simulink model "prescan_repl1"  (R2019a)
settings: Solver=VariableStepAuto  StartTime=0.0  StopTime=10.0  RelTol=1e-3  EnableMultiTasking=on
libraries: ProSivic_Sensors x4, ProSivic_Commands x2
settings Model: Creator=PGS  LastModifiedBy=Markus Borg
settings DataIOCC: ReturnWorkspaceOutputs=off
settings OptimizationCC: LifeSpan=inf
settings DebuggingCC: SFUnexpectedBacktrackingDiag=warning  SFNoUnconditionalDefaultTransitionDiag=warning  ArithmeticOperatorsInVariantConditions=warning
settings SFSimCC: SimUseLocalCustomCode=off
settings RTWCC: RTWUseLocalCustomCode=off
settings CodeAppCC: StateflowObjectComments=on
settings GRTTargetCC: TargetLangStandard=C89/C90 (ANSI)  GeneratePreprocessorConditionals=Disable all
settings ConfigComp: CovMetricSettings=dw  CovHtmlReporting=on  CovSaveCumulativeToWorkspaceVar=on  CovSaveSingleToWorkspaceVar=on  CovExternalEMLEnable=off

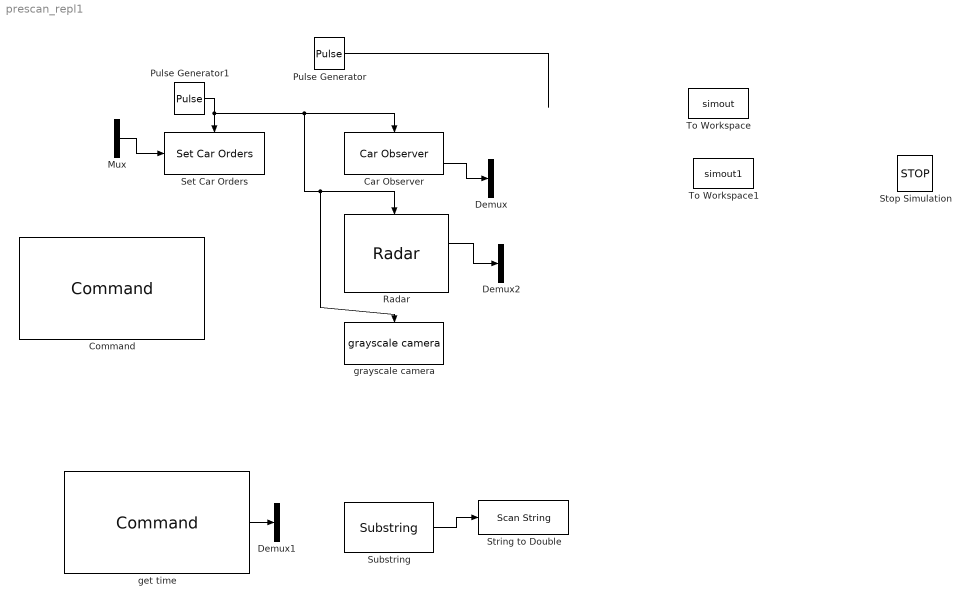
== system prescan_repl1 ==
  " grayscale camera" : ProSivic_Sensors/ grayscale camera  topic=camera/cam  h=480  w=752  color=off
  Car Observer : ProSivic_Sensors/Car Observer  SystemSampleTime=-1
  Command : ProSivic_Commands/Command  command=new sivicTime timeWrapper1  ip=localhost
  Demux : Demux  Outputs=2
  Demux1 : Demux  Outputs=2
  Demux2 : Demux  Outputs=2
  Mux : Mux  Inputs=2
  Pulse Generator : DiscretePulseGenerator  PulseType=Time based  Period=0.5  PulseWidth=5
  Pulse Generator1 : DiscretePulseGenerator  PulseType=Time based  Period=0.005  PulseWidth=5
  Radar : ProSivic_Sensors/Radar  Description=Radar block retreives the latest radar information from the ProSiVIC DDS store.  SystemSampleTime=-1
  Set Car Orders : ProSivic_Sensors/Set Car Orders  topic=Vehicle/car
  Stop Simulation : Stop
  String to Double : ScanString  Format="\"%lf\""
  Substring : Substring
  To Workspace : ToWorkspace  VariableName=simout  SaveFormat=Timeseries  SampleTime=-1
  To Workspace1 : ToWorkspace  VariableName=simout1  SaveFormat=Timeseries  SampleTime=-1
  get time : ProSivic_Commands/Command  command=GETP timeWrapper6 SimuTime  ip=localhost
  wires:
  Pulse Generator/1 -> ?
  ? -> To Workspace/1
  ? -> To Workspace1/1
  Car Observer/2 -> Demux/1
  Mux/1 -> Set Car Orders/1
  Pulse Generator1/1 -> " grayscale camera"/Trigger, Radar/Trigger, Car Observer/Trigger, Set Car Orders/Trigger
  Substring/1 -> String to Double/1
  get time/1 -> Demux1/1
  Radar/2 -> Demux2/1
